simulink library "lib_DCDCManager"  (R2017a)
settings: Solver=VariableStepAuto  StartTime=0.0  StopTime=10.0  RelTol=1e-3
libraries: simulink x1
settings Model: Creator=Di Russo  LastModifiedBy=Vraj M

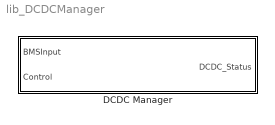
== system lib_DCDCManager ==
  DCDC Manager : Subsystem

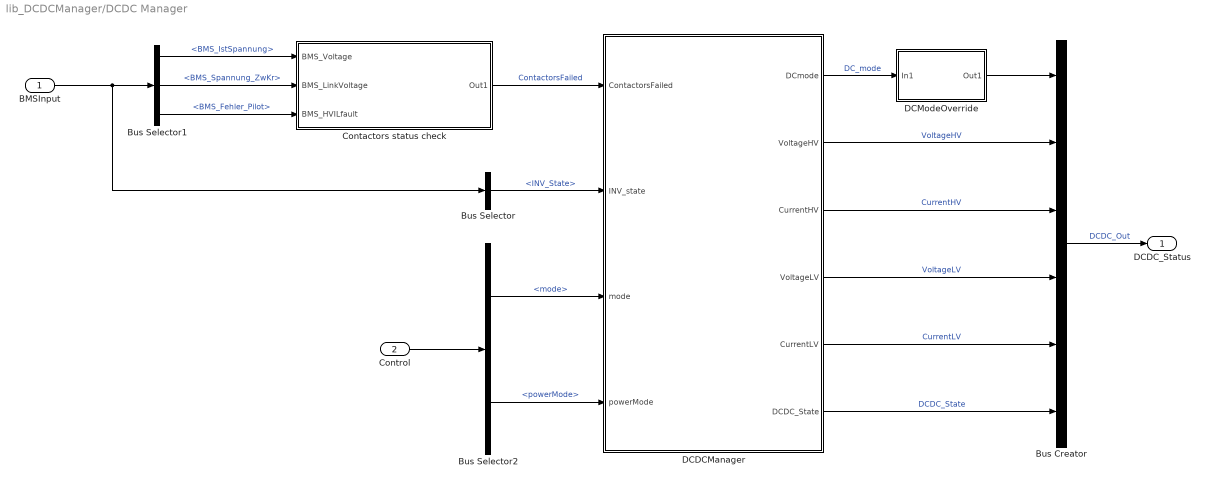
== system lib_DCDCManager/DCDC Manager ==
  BMSInput : Inport
  Control : Inport  Port=2
  Bus Creator : BusCreator  Inputs=6
  Bus Selector : BusSelector  OutputSignals=from_CAN.fromHV_CAN.from_MCU.INV_VCU_01.INV_State
  Bus Selector1 : BusSelector  OutputSignals=from_CAN.fromHV_CAN.from_BMSHybrid.BMS_HYB_02.BMS_IstSpannung,from_CAN.fromHV_CAN.from_BMSHybrid.BMS_Spannung_ZwKr,from_CAN.fromHV_CAN.from_BMSHybrid.BMS_HYB_02.BMS_Fehler_Pilot
  Bus Selector2 : BusSelector  OutputSignals=mode,powerMode
  Contactors status check : Subsystem
  DCDCManager : Stateflow chart  RequirementInfo={} %GIDa_0406d6c1_ee5b_4673_84b2_b23717c96a9a  TreatAsAtomicUnit=on
  DCModeOverride : Subsystem
  DCDC_Status : Outport
  wires:
  DCModeOverride/1(Out1) -> Bus Creator/1
  DCDCManager/1(DCmode) -> DCModeOverride/1(In1)  "DC_mode"
  Bus Selector2/2 -> DCDCManager/4(powerMode)  "<powerMode>"
  Control/1 -> Bus Selector2/1
  Bus Selector2/1 -> DCDCManager/3(mode)  "<mode>"
  DCDCManager/6(DCDC_State) -> Bus Creator/6  "DCDC_State"
  Bus Creator/1 -> DCDC_Status/1  "DCDC_Out"
  DCDCManager/2(VoltageHV) -> Bus Creator/2  "VoltageHV"
  DCDCManager/3(CurrentHV) -> Bus Creator/3  "CurrentHV"
  DCDCManager/4(VoltageLV) -> Bus Creator/4  "VoltageLV"
  DCDCManager/5(CurrentLV) -> Bus Creator/5  "CurrentLV"
  Bus Selector/1 -> DCDCManager/2(INV_state)  "<INV_State>"
  Contactors status check/1(Out1) -> DCDCManager/1(ContactorsFailed)  "ContactorsFailed"
  Bus Selector1/2 -> Contactors status check/2(BMS_LinkVoltage)  "<BMS_Spannung_ZwKr>"
  Bus Selector1/3 -> Contactors status check/3(BMS_HVILfault)  "<BMS_Fehler_Pilot>"
  Bus Selector1/1 -> Contactors status check/1(BMS_Voltage)  "<BMS_IstSpannung>"
  BMSInput/1 -> Bus Selector1/1, Bus Selector/1

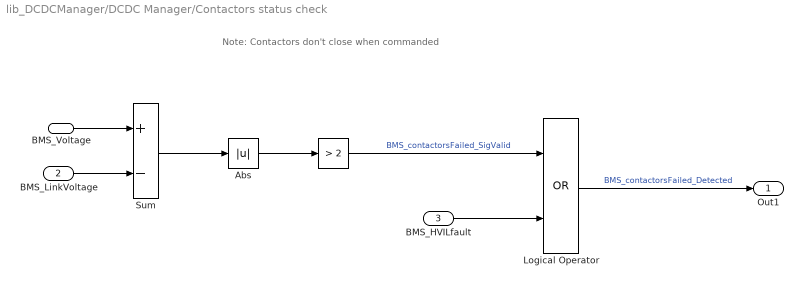
== system lib_DCDCManager/DCDC Manager/Contactors status check ==
  note: Note: Contactors don't close when commanded
  BMS_Voltage : Inport
  BMS_LinkVoltage : Inport  Port=2
  BMS_HVILfault : Inport  Port=3
  " " : simulink/Logic and Bit Operations/Compare To Constant  relop=>  const=2  OutDataTypeStr=boolean
  Abs : Abs
  Logical Operator : Logic  Operator=OR  AllPortsSameDT=off  OutDataTypeStr=boolean
  Sum : Sum  Inputs=+-
  Out1 : Outport
  wires:
  " "/1 -> Logical Operator/1  "BMS_contactorsFailed_SigValid"
  BMS_HVILfault/1 -> Logical Operator/2
  BMS_LinkVoltage/1 -> Sum/2
  Abs/1 -> " "/1
  Sum/1 -> Abs/1
  Logical Operator/1 -> Out1/1  "BMS_contactorsFailed_Detected"
  BMS_Voltage/1 -> Sum/1

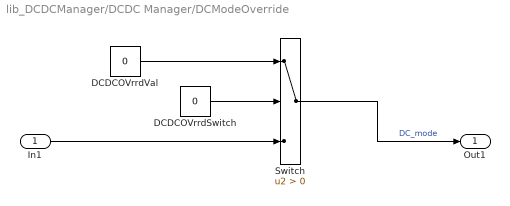
== system lib_DCDCManager/DCDC Manager/DCModeOverride ==
  In1 : Inport
  DCDCOVrrdSwitch : Constant  Value=0
  DCDCOVrrdVal : Constant  Value=0
  Switch : Switch  Criteria=u2 > Threshold
  Out1 : Outport
  wires:
  DCDCOVrrdVal/1 -> Switch/1
  DCDCOVrrdSwitch/1 -> Switch/2
  In1/1 -> Switch/3
  Switch/1 -> Out1/1  "DC_mode"

== stateflow chart lib_DCDCManager/DCDC Manager/DCDCManager ==
  state DCDC_Initialization
    state Initialization
      entry: DCDC_State = 1;
    state Power_On
      entry: DCmode = 1;
      DCDC_State = 2;
      VoltageHV = 0;
      VoltageLV =14;
      CurrentHV = 20;
      CurrentLV = 173;
    (default) -> Initialization
    Initialization -> Power_On : [ContactorsFailed == 0]
  state Delay
  state DCDC_Off
    entry: DCDC_State = 4;
    DCmode = 0;
  (default) -> DCDC_Initialization
  Delay -> DCDC_Initialization : after(5,sec)
  DCDC_Initialization -> DCDC_Off : [INV_state == 14 || ...
      | ContactorsFailed == 1|| ...
      | mode == 7]
  DCDC_Off -> Delay : [(INV_state == 3 || INV_state == 8) && ...
      | ContactorsFailed == 0&&...
      |  (powerMode ==1|| powerMode == 2 || powerMode == 3)]
  data: ContactorsFailed input; DCmode output; VoltageHV output; CurrentHV output; VoltageLV output; CurrentLV output; INV_state input; DCDC_State output; mode input; powerMode input
